simulink model "rdt"  (R2024b)
settings: Solver=FixedStepDiscrete  StartTime=0.0  StopTime=1  FixedStep=0.1  RelTol=1e-3
model workspace (MAT data in the model file):
  input = Simulink.Bus
  input.Alignment = -1
  input.PreserveElementDimensions = 0
  input.Elements_internal = Simulink.BusElement
  input.Elements_internal.DimensionsMode = 'Fixed'
  input.Elements_internal.SamplingMode = 'Sample based'
  input.Elements_internal.SampleTime = -1
  input.Elements_internal.Name = 'data'
  input.Elements_internal.DataType_internal = 'uint8'
  input.Elements_internal.Complexity = 'real'
  input.Elements_internal.Dimensions = 1
  input.DataScope = 'Auto'
  output = Simulink.Bus
  output.Alignment = -1
  output.PreserveElementDimensions = 0
  output.Elements_internal = Simulink.BusElement
  output.Elements_internal.DimensionsMode = 'Fixed'
  output.Elements_internal.SamplingMode = 'Sample based'
  output.Elements_internal.SampleTime = -1
  output.Elements_internal.Name = 'data'
  output.Elements_internal.DataType_internal = 'uint8'
  output.Elements_internal.Complexity = 'real'
  output.Elements_internal.Dimensions = 1
  output.DataScope = 'Auto'
libraries: dspnetwork x4, simulink x2, spsEdgeDetectorLib x1
settings Model: Creator=Amin  LastModifiedBy=Amin

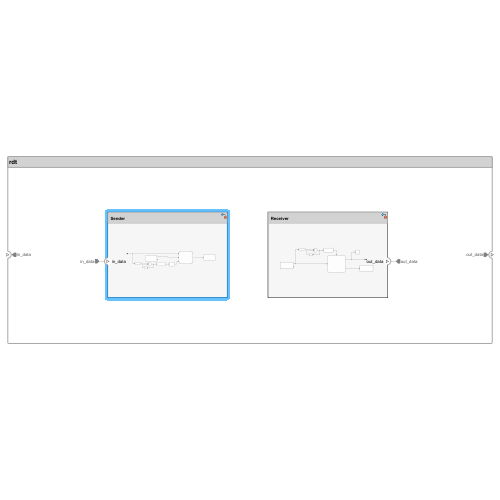
[thumbnail: Simulink's stored preview of the top-level diagram]
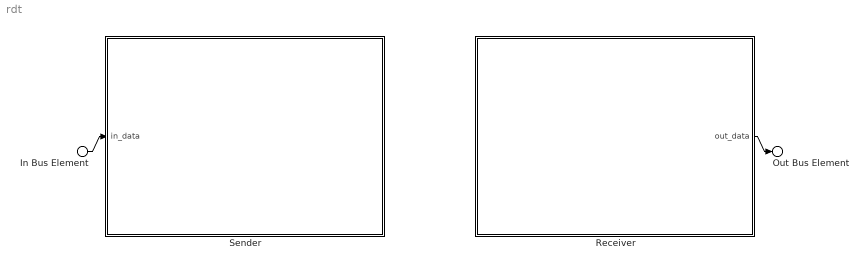
== system rdt ==
  In Bus Element : Inport  PortName=in_data
  Receiver : Subsystem
      settings: PortSchema="{\"entries\":[{\"content\":{\"headerSize\":26,\"margin\":15,\"minimumSpacing\":25,\"sides\":[{\"content\":{},\"type\":\"ConnectorPlacement.EquallySpacedRectSide\",\"uuid\":\"fc03e76e-2688-4f9e-bb8a-0bf1b636fd8d\"},{\"content\":{\"connectorIds\":[\"Out1\"],\"side\":\"RIGHT\"},\"type\":\"ConnectorPlacement.EquallySpacedRectSide\",\"uuid\":\"b7f372b2-e80c-40ec-aab5-1d265ad8a23a\"},{\"content\":{\"side\":\"TOP\"},\"type\":\"ConnectorPlacement.EquallySpacedRectSide\",\"uuid\":\"9fb0d473-dbe2-43fe-8153-a1c1b7fed0d9\"}]},\"type\":\"ConnectorPlacement.EquallySpacedConnector\",\"uuid\":\"3e655b9b-c4b3-4b1e-b65d-35ded5f10b13\"}],\"packageUris\":[\"http://schema.mathworks.com/mf0/Connector/R2020b\"],\"version\":\"1.0\"}"
  Sender : Subsystem
      settings: PortSchema="{\"entries\":[{\"content\":{\"headerSize\":26,\"margin\":15,\"minimumSpacing\":25,\"sides\":[{\"content\":{\"connectorIds\":[\"In1\"]},\"type\":\"ConnectorPlacement.EquallySpacedRectSide\",\"uuid\":\"fc03e76e-2688-4f9e-bb8a-0bf1b636fd8d\"},{\"content\":{\"side\":\"RIGHT\"},\"type\":\"ConnectorPlacement.EquallySpacedRectSide\",\"uuid\":\"b7f372b2-e80c-40ec-aab5-1d265ad8a23a\"},{\"content\":{\"side\":\"TOP\"},\"type\":\"ConnectorPlacement.EquallySpacedRectSide\",\"uuid\":\"9fb0d473-dbe2-43fe-8153-a1c1b7fed0d9\"}]},\"type\":\"ConnectorPlacement.EquallySpacedConnector\",\"uuid\":\"3e655b9b-c4b3-4b1e-b65d-35ded5f10b13\"}],\"packageUris\":[\"http://schema.mathworks.com/mf0/Connector/R2020b\"],\"version\":\"1.0\"}"
  Out Bus Element : Outport  PortName=out_data
  wires:
  In Bus Element/1 -> Sender/1(in_data)
  Receiver/1(out_data) -> Out Bus Element/1

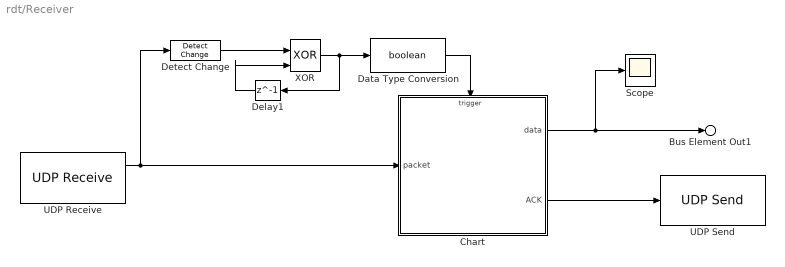
== system rdt/Receiver ==
  Chart : Stateflow chart  TreatAsAtomicUnit=on
  Data Type Conversion : DataTypeConversion  OutDataTypeStr=boolean  SaturateOnIntegerOverflow=off  RndMeth=Floor
  Delay1 : Delay  DelayLength=1
  Detect Change : simulink/Logic and Bit Operations/Detect Change  vinit=0  OutDataTypeStr=uint8
  Scope : Scope
  UDP Receive : dspnetwork/UDP Receive  localURL='0.0.0.0'  localPort=25000  remoteURL='127.0.0.1'  remotePort=-1  recvBufferSize=8192  dims=1  signalDatatype=uint16  isComplex=off  isVarSize=off  showBlockingTime=off  blockingTime=0  sampletime=0.1  blockPlatform=[]
      settings: LibrarySourceBlock=dspsrcs4/UDP Receive
  UDP Send : dspnetwork/UDP Send  remoteURL='127.0.0.1'  remotePort=26000  localURL='0.0.0.0'  localPortSource=Automatically determine  localPort=-1  sendBufferSize=8192  sampletime=-1  blockPlatform=[]  separateLengthPort=0
      settings: LibrarySourceBlock=dspsnks4/UDP Send
  XOR : Logic  Operator=XOR  IconShape=distinctive  AllPortsSameDT=off  OutDataTypeStr=boolean
  Bus Element Out1 : Outport  PortName=out_data  Element=data
  wires:
  Detect Change/1 -> XOR/1
  XOR/1 -> Delay1/1, Data Type Conversion/1
  Chart/2(ACK) -> UDP Send/1
  Chart/1(data) -> Scope/1, Bus Element Out1/1
  Delay1/1 -> XOR/2
  UDP Receive/1 -> Chart/1("packet "), Detect Change/1
  Data Type Conversion/1 -> Chart/Trigger

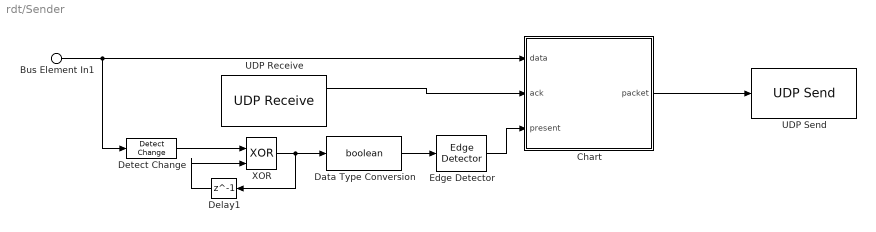
== system rdt/Sender ==
  Bus Element In1 : Inport  PortName=in_data  Element=data
  Chart : Stateflow chart  TreatAsAtomicUnit=on
  Data Type Conversion : DataTypeConversion  OutDataTypeStr=boolean  SaturateOnIntegerOverflow=off  RndMeth=Floor
  Delay1 : Delay  DelayLength=1
  Detect Change : simulink/Logic and Bit Operations/Detect Change  vinit=0  OutDataTypeStr=uint8
  Edge Detector : spsEdgeDetectorLib/Edge Detector  model=Either  ic=0  Ts=0
      settings: LibrarySourceBlock=sps_lib/Control/Edge Detector
  UDP Receive : dspnetwork/UDP Receive  localURL='0.0.0.0'  localPort=26000  remoteURL='127.0.0.1'  remotePort=-1  recvBufferSize=8192  dims=1  signalDatatype=single  isComplex=off  isVarSize=off  showBlockingTime=off  blockingTime=0  sampletime=0.1  blockPlatform=[]
      settings: LibrarySourceBlock=dspsrcs4/UDP Receive
  UDP Send : dspnetwork/UDP Send  remoteURL='127.0.0.1'  remotePort=25000  localURL='0.0.0.0'  localPortSource=Automatically determine  localPort=-1  sendBufferSize=8192  sampletime=-1  blockPlatform=[]  separateLengthPort=0
      settings: LibrarySourceBlock=dspsnks4/UDP Send
  XOR : Logic  Operator=XOR  IconShape=distinctive  AllPortsSameDT=off  OutDataTypeStr=boolean
  wires:
  Detect Change/1 -> XOR/1
  XOR/1 -> Delay1/1, Data Type Conversion/1
  Delay1/1 -> XOR/2
  Data Type Conversion/1 -> Edge Detector/1
  Edge Detector/1 -> Chart/3(present)
  UDP Receive/1 -> Chart/2(ack)
  Chart/1(packet) -> UDP Send/1
  Bus Element In1/1 -> Chart/1(data), Detect Change/1

== stateflow chart rdt/Receiver/Chart ==
  settings: executeAtInitialization=1
  state Wait_for_1_from_below
  state Wait_for_0_from_below1
  (default) -> Wait_for_1_from_below
  Wait_for_1_from_below -> Wait_for_0_from_below1 : [packetEvent && check_packet(packet)]{[data, ACK] = send_data_ack(packet, ACK)}
  Wait_for_0_from_below1 -> Wait_for_1_from_below : [packetEvent && check_packet(packet)]{[data, ACK] = send_data_ack(packet, ACK)}
  data: f function_output; p function_input; value function_input; header function_output; polynomial function_input; p function_input; d function_output; a function_input; a function_output; data output uint8 =0; packet input uint16; ACK output single =0
  events: packetEvent input EITHER_EDGE_EVENT
  function f = check_packet(p):
    | function f = check_packet(p)
    | 
    |     header = uint8(bitshift(p, -8));
    |     raw_data = uint8(bitand(p, 0x00FF));
    |     if crc4(raw_data, 19) == header
    |         f = true;
    |     else
    |         f = false;
    |     end
    |     
    | end
  function header = crc4(value, polynomial):
    | function header = crc4(value, polynomial)
    |         
    |     % Initialize the CRC register to 0
    |     crc = uint8(0);
    |         
    |     % Loop over each bit in the input byte (MSB first)
    |     for i = 7:-1:-4
    |         % XOR the MSB of the input with the MSB of the CRC register
    |         crc = bitxor(crc, bitand(bitshift(value, -i), 1));  % Shift input and XOR
    |             
    |         % If the MSB of the CRC is 1, perform the polynomial division (XOR)
    |         if bitget(crc, 5)  % Check if MSB (bit 5) of 8-bit crc is set
    |            crc = bitxor(crc, polynomial);  % Perform division by XOR with polynomial
    |         end
    |             
    |         if i ~= -4
    |             % Shift CRC register left by 1 bit
    |             crc = bitshift(crc, 1);
    |         end
    |     end
    |         
    |     
    |     % Final CRC value is the remainder in the lowest 4 bits
    |     header = bitand(crc, 15);  % Mask to get the lower 4 bits as the CRC result
    | end
  function [d, a] = send_data_ack(p, a):
    | function [d, a] = send_data_ack(p, a)
    | 
    |     d = uint8(bitand(p, 0x0011));
    |     
    |     if a == single(0)
    |         a = single(1);
    |     else
    |         a = single(0);
    |     end
    | end

== stateflow chart rdt/Sender/Chart ==
  state Wait_for_call_1_from_above
  state Wait_for_ACK1
  state Wait_for_call_0_from_above
  state Wait_for_ACK0
  Wait_for_ACK1 -> Wait_for_ACK1 [order 3] : [after(TIMEOUT, sec)]{packet = uint16(calculation(data));}
  (default) -> Wait_for_call_1_from_above
  Wait_for_call_1_from_above -> Wait_for_call_1_from_above [order 2] : [ack==1]
  Wait_for_ACK1 -> Wait_for_ACK1 [order 2] : [ack==0]
  Wait_for_call_1_from_above -> Wait_for_ACK1 [order 1] : [present==1]{packet=uint16(calculation(data))}
  Wait_for_call_0_from_above -> Wait_for_call_1_from_above [order 1] : [ack==0]
  Wait_for_ACK1 -> Wait_for_ACK0 [order 1] : [ack==1]
  Wait_for_call_0_from_above -> Wait_for_call_0_from_above [order 2] : [ack==0]
  Wait_for_ACK0 -> Wait_for_ACK0 [order 2] : [ack==1]
  Wait_for_ACK0 -> Wait_for_call_0_from_above [order 1] : [present==1]{packet=uint16(calculation(data))}
  Wait_for_call_0_from_above -> Wait_for_call_0_from_above [order 3] : [after(TIMEOUT, sec)]{packet = uint16(calculation(data));}
  data: value function_input; header function_output; polynomial function_input; input function_input uint8; output function_output uint16; data input uint8; ack input single; present input boolean; packet output uint16; TIMEOUT constant double =4
  function header = crc4(value, polynomial):
    | function header = crc4(value, polynomial)
    |         
    |     % Initialize the CRC register to 0
    |     crc = uint8(0);
    |         
    |     % Loop over each bit in the input byte (MSB first)
    |     for i = 7:-1:-4
    |         % XOR the MSB of the input with the MSB of the CRC register
    |         crc = bitxor(crc, bitand(bitshift(value, -i), 1));  % Shift input and XOR
    |             
    |         % If the MSB of the CRC is 1, perform the polynomial division (XOR)
    |         if bitget(crc, 5)  % Check if MSB (bit 5) of 8-bit crc is set
    |            crc = bitxor(crc, polynomial);  % Perform division by XOR with polynomial
    |         end
    |             
    |         if i ~= -4
    |             % Shift CRC register left by 1 bit
    |             crc = bitshift(crc, 1);
    |         end
    |     end
    |         
    |     
    |     % Final CRC value is the remainder in the lowest 4 bits
    |     header = bitand(crc, 15);  % Mask to get the lower 4 bits as the CRC result
    | end
  function output = calculation(input):
    | function output = calculation(input)
    | 
    |     output = bitor(uint16(input), bitshift(uint16(crc4(input, 19)), 8));
    | 
    | end
